simulink model "tf7"  (R2024a)
settings: Solver=VariableStepAuto  StartTime=0.0  StopTime=10.0  RelTol=1e-3
settings Model: Creator=tusha  LastModifiedBy=tusha

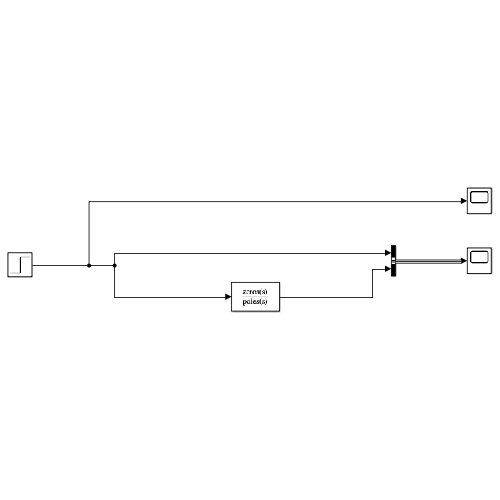
[thumbnail: Simulink's stored preview of the top-level diagram]
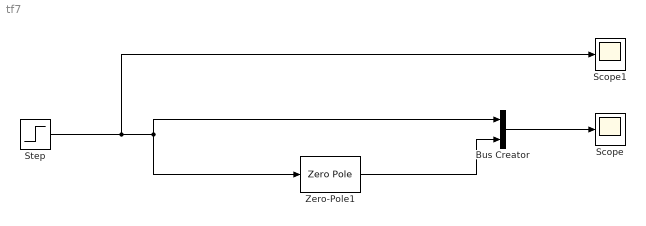
== system tf7 ==
  Bus Creator : BusCreator  Inputs=2
  Scope : Scope
  Scope1 : Scope
  Step : Step  SampleTime=0
  Zero-Pole1 : ZeroPole  Zeros=[3]  Poles=[2 2+3i 2-3i]  Gain=[10]
  wires:
  Zero-Pole1/1 -> Bus Creator/2
  Step/1 -> Scope1/1, Bus Creator/1, Zero-Pole1/1
  Bus Creator/1 -> Scope/1
